simulink model "latestMPCforRTMapsGen"  (R2024a)
settings: Solver=FixedStepDiscrete  StartTime=0  StopTime=100  FixedStep=.05  RelTol=1e-3
undefined symbols (not defined in the file or in its folder): act_t_delay, aero_const, delta_U_max, delta_U_min, driver_set_spd, m, N, Qbar, Rbar, simStepSize, U_max, U_min, y_max, Y_min
settings Model: PacingRate=10  Creator=darkh  LastModifiedBy=darkh
settings DataIOCC: ReturnWorkspaceOutputsName=sltest_internal_rrSimulationOutputVariable
settings OptimizationCC: ZeroExternalMemoryAtStartup=off  ZeroInternalMemoryAtStartup=off
settings DebuggingCC: AlgebraicLoopMsg=none
settings RTWCC: Description=Generate an RTMaps component embedding the model  SystemTargetFile=rtmaps.tlc  TemplateMakefile=rtmaps_default_tmf  PostCodeGenCommand=rtmaps_post_code_generation(buildInfo)  RetainRTWFile=on  TargetLang=C++  GPUComputeCapability=3.5
settings STFCustomTargetCC: TargetLangStandard=C++11 (ISO)  ModelReferenceCompliant=off  ConcurrentExecutionCompliant=on  CombineOutputUpdateFcns=on  CodeInterfacePackaging=C++ class  CPPClassGenCompliant=on  GRTInterface=off  UseToolchainInfoCompliant=off  SystemTargetFile=rtmaps.tlc
settings GRTTargetCC: TargetLangStandard=C++11 (ISO)  ModelReferenceCompliant=off  ParMdlRefBuildCompliant=off  CompOptLevelCompliant=off  MatFileLogging=off  CodeInterfacePackaging=C++ class  UseToolchainInfoCompliant=off
settings ConfigComp: CovSaveName=sltest_covdata  CovMetricSettings=dcmwe  CovEnableCumulative=off  CovSaveSingleToWorkspaceVar=on  CovSaveOutputData=off

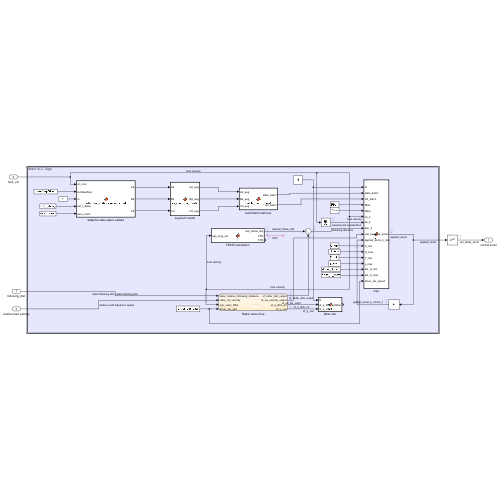
[thumbnail: Simulink's stored preview of the top-level diagram]
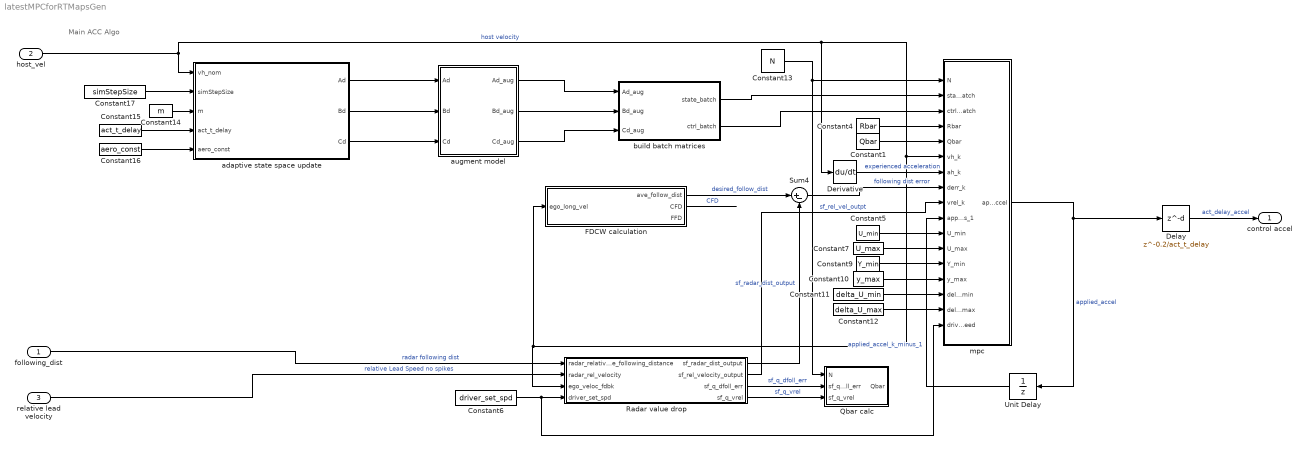
== system latestMPCforRTMapsGen ==
  note: Main ACC Algo
  following_dist : Inport
  host_vel : Inport  Port=2
  relative lead velocity : Inport  Port=3
  Constant1 : Constant  Value=Qbar
  Constant10 : Constant  Value=y_max
  Constant11 : Constant  Value=delta_U_min
  Constant12 : Constant  Value=delta_U_max
  Constant13 : Constant  Value=N
  Constant14 : Constant  Value=m
  Constant15 : Constant  Value=act_t_delay
  Constant16 : Constant  Value=aero_const
  Constant17 : Constant  Value=simStepSize
  Constant4 : Constant  Value=Rbar
  Constant5 : Constant  Value=U_min
  Constant6 : Constant  Value=driver_set_spd
  Constant7 : Constant  Value=U_max
  Constant9 : Constant  Value=Y_min
  Delay : Delay  DelayLength=0.2/act_t_delay
  Derivative : Derivative
  FDCW calculation : MATLAB Function  TreatAsAtomicUnit=on
  Qbar calc : MATLAB Function  TreatAsAtomicUnit=on  SystemSampleTime=simStepSize
  Radar value drop : Stateflow chart  TreatAsAtomicUnit=on
  Sum4 : Sum  Inputs=|+-
  Unit Delay : UnitDelay  SampleTime=-1  HasFrameUpgradeWarning=on
  adaptive state space update : MATLAB Function  TreatAsAtomicUnit=on
  augment model : MATLAB Function  TreatAsAtomicUnit=on
  build batch matrices : MATLAB Function  TreatAsAtomicUnit=on  SystemSampleTime=simStepSize
  mpc : MATLAB Function  TreatAsAtomicUnit=on  SystemSampleTime=simStepSize
  control accel : Outport
  wires:
  host_vel/1 -> adaptive state space update/1(vh_nom), Derivative/1, FDCW calculation/1(ego_long_vel), Radar value drop/3(ego_veloc_fdbk), mpc/6(vh_k)  "host velocity"
  Sum4/1 -> mpc/8(derr_k)  "following dist error"
  relative lead velocity/1 -> Radar value drop/2(radar_rel_velocity)  "relative Lead Speed no spikes"
  FDCW calculation/1(ave_follow_dist) -> Sum4/1  "desired_follow_dist"
  FDCW calculation/2(CFD) -> ?  "CFD"
  following_dist/1 -> Radar value drop/1(radar_relative_following_distance)  "radar following dist"
  Derivative/1 -> mpc/7(ah_k)  "experienced acceleration"
  Constant4/1 -> mpc/4(Rbar)
  Radar value drop/1(sf_radar_dist_output) -> Sum4/2  "sf_radar_dist_output"
  Constant6/1 -> mpc/17(driver_set_speed), Radar value drop/4(driver_set_spd)
  Radar value drop/2(sf_rel_velocity_output) -> mpc/9(vrel_k)  "sf_rel_vel_outpt"
  Radar value drop/3(sf_q_dfoll_err) -> Qbar calc/2(sf_q_dfoll_err)  "sf_q_dfoll_err"
  Radar value drop/4(sf_q_vrel) -> Qbar calc/3(sf_q_vrel)  "sf_q_vrel"
  Unit Delay/1 -> mpc/10(applied_accel_k_minus_1)  "applied_accel_k_minus_1"
  Constant5/1 -> mpc/11(U_min)
  Constant7/1 -> mpc/12(U_max)
  Constant9/1 -> mpc/13(Y_min)
  Constant10/1 -> mpc/14(y_max)
  Constant11/1 -> mpc/15(del_U_min)
  Constant12/1 -> mpc/16(del_U_max)
  Constant1/1 -> mpc/5(Qbar)
  mpc/1(applied_accel) -> Unit Delay/1, Delay/1  "applied_accel"
  Constant14/1 -> adaptive state space update/3(m)
  Constant15/1 -> adaptive state space update/4(act_t_delay)
  Constant16/1 -> adaptive state space update/5(aero_const)
  Constant17/1 -> adaptive state space update/2(simStepSize)
  augment model/3(Cd_aug) -> build batch matrices/3(Cd_aug)
  augment model/2(Bd_aug) -> build batch matrices/2(Bd_aug)
  augment model/1(Ad_aug) -> build batch matrices/1(Ad_aug)
  Constant13/1 -> Qbar calc/1(N), mpc/1(N)
  adaptive state space update/1(Ad) -> augment model/1(Ad)
  adaptive state space update/2(Bd) -> augment model/2(Bd)
  adaptive state space update/3(Cd) -> augment model/3(Cd)
  Delay/1 -> control accel/1  "act_delay_accel"
  build batch matrices/1(state_batch) -> mpc/2(state_batch)
  build batch matrices/2(ctrl_batch) -> mpc/3(ctrl_batch)

== matlab function latestMPCforRTMapsGen/build batch matrices ==
  data: state_batch output; Ad_aug input; Bd_aug input; Cd_aug input; ctrl_batch output
function [state_batch,ctrl_batch] = batch_matrix_build(Ad_aug,Bd_aug,Cd_aug)
[ny1,ny2] = size(Cd_aug);
[~,nu] = size(Bd_aug);

N=20;

% Building batch matrices for MPC prediction of output states
% batch matrix for state vector
state_batch = zeros(N*ny1, ny2);
for i = 1:N
    state_batch((i-1)*ny1+1 : i*ny1, :) = Cd_aug*(Ad_aug^i);
end

% Batch matrix for control vector
ctrl_batch = zeros(N*ny1, N*nu); % pre-allocate, fixed size

Apow = eye(size(Ad_aug)); % A^0
for i = 1:N
    % first column block for row i
    ctrl_batch((i-1)*ny1+(1:ny1), 1:nu) = Cd_aug*Apow*Bd_aug;
    % copy to the right for j = 2…i
    col = nu; % offset for next column
    Apow_j = Apow;
    for j = 2:i
        Apow_j = Apow_j / Ad_aug; % A^(i-j) (cheaper than repeated power)
        ctrl_batch((i-1)*ny1+(1:ny1), (j-1)*nu+(1:nu)) = Cd_aug*Apow_j*Bd_aug;
        col = col + nu;
    end
    Apow = Apow*Ad_aug; % advance A^i
end

== matlab function latestMPCforRTMapsGen/FDCW calculation ==
  settings: updateMethod=DISCRETE
  data: ego_long_vel input; ave_follow_dist output; CFD output; FFD output
% Function to determine the closest (CFD) and furthest follow distance (FFD) for the
% ego vehicle relative to the lead vehicle given the ego vehicle's current
% velocity

% This function outputs the middle distance value between the CFD and FFD
% and those values respectively as well

function [ave_follow_dist, CFD, FFD] = fcn(ego_long_vel)
    persistent dist_history window_size smoothing_weights
    
    % Initialize (first call only)
    if isempty(dist_history)
        window_size = 5;  % Number of past samples
        dist_history = zeros(1, window_size);
        
        % Define and normalize weights (e.g., linear decay)
        smoothing_weights = linspace(1, 0.5, window_size);  % Weights from 1.0 to 0.5
        smoothing_weights = smoothing_weights / sum(smoothing_weights);  % Normalize
    end
    ego_long_vel_mph = ego_long_vel*2.23694;
    
    if ego_long_vel_mph > 0 && ego_long_vel_mph < 20
        CFD = 2.8*ego_long_vel_mph^0.45+8;
        FFD = 100-0.2*(20-ego_long_vel_mph)^2;
    elseif ego_long_vel_mph <= 0
        CFD = 8;
        FFD = 100-0.2*(20)^2;
    else
        CFD = 2.8*ego_long_vel_mph^0.45+8;
        FFD = 100;
    end
    AveFollowDist_Gain = 3;


    % --- Update history buffer ---
    dist_history = [ ((AveFollowDist_Gain-1)*CFD + FFD)/AveFollowDist_Gain , dist_history(1:end-1)];  % FIFO

    % --- Smoothed average (weighted, normalized) ---
    smoothed_ave_dist = sum(dist_history .* smoothing_weights);
    
    % --- Clamp to CFD/FFD bounds ---
    ave_follow_dist = min(max(smoothed_ave_dist, CFD), FFD);
end

== matlab function latestMPCforRTMapsGen/adaptive state space update ==
  data: vh_nom input; simStepSize input; Ad output; m input; act_t_delay input; aero_const input; Bd output; Cd output
function [Ad,Bd,Cd] = adaptive_state_space_model(vh_nom, simStepSize, m, act_t_delay, aero_const)
% multiplying A matrix term with current vehicle velocity vh_nom to update
% state space model for adaptive MPC
Ac = [0,1,0,0; -aero_const*vh_nom/(m*act_t_delay), -1/act_t_delay, 0,0;0,0,0,-1;0,-1,0,0]; % with drag term
% Ac = [0,1,0,0; 0, -1/act_t_delay, 0,0;0,0,0,-1;0,-1,0,0]; % without the velocity dependent drag term
Bc = [0;1/act_t_delay;0;0];

% Using Euler discretization to obtain the discrete time matrices from the continuous time system
Ad = eye(4) + Ac.*simStepSize;
Bd = Bc.*simStepSize;
Cd = eye(4);

== matlab function latestMPCforRTMapsGen/mpc ==
  data: N input; state_batch input; ctrl_batch input; Rbar input; Qbar input; applied_accel output; vh_k input; ah_k input; derr_k input; vrel_k input; applied_accel_k_minus_1 input; U_min input; U_max input; Y_min input; y_max input; del_U_min input; del_U_max input; driver_set_speed input
function applied_accel  = mpc(N, state_batch, ctrl_batch, Rbar, Qbar, vh_k, ah_k, derr_k, vrel_k, applied_accel_k_minus_1, U_min, U_max, Y_min, y_max, del_U_min, del_U_max, driver_set_speed)
% Defining MPC and system variables
num_outpts = 4
num_ctrl = 1;

state_vec_curr = [vh_k, ah_k, derr_k, vrel_k, applied_accel_k_minus_1]';

H = 2*(ctrl_batch' * Qbar * ctrl_batch + Rbar); % symmetric Hessian
% tiny regulariser to ensure positive-definite
H = (H+H.')/2 + 1e-8*eye(size(H));

f = 2*(ctrl_batch' * Qbar * state_batch * state_vec_curr);

persistent del_Uopt_k_minus_1 % defining persistent variable to keep track of computed optimal control signal from previous iteration
if isempty(del_Uopt_k_minus_1)
    % del_Uopt_k_minus_1 = [0,0,0,0,0,0,0,0,0,0]'; % for N = 10
    del_Uopt_k_minus_1 = [0,0,0,0,0,0,0,0,0,0,0,0,0,0,0,0,0,0,0,0]'; % for N = 20
end

%% Defining the control input limits on delta_u based on limits on u

% Determining U(k-1) from the previous control signal u(k-1) and the previous full predicted control signal delta_Uopt(k-1)
Ubar_k_minus_1 = zeros(N*num_ctrl, 1); % Initializing
Ubar_k_minus_1(1:num_ctrl,:) = applied_accel_k_minus_1; % Populating the first control vector in Uopt(k-1) as u(k-1) = [accel_app(k-1)]'

for i = 1:N-1
    Ubar_k_minus_1(i*num_ctrl+1 : (i+1)*num_ctrl, :) = Ubar_k_minus_1((i-1)*num_ctrl+1 : i*num_ctrl, :) + del_Uopt_k_minus_1(i*num_ctrl+1 : (i+1)*num_ctrl, :); % performing u(k) = u(k-1) + delta_u(k-1) for all elements to populate Uopt(k-1)
end

% Defining the maximum output limit Y_max since the driver set speed may change
Y_max = zeros(N*num_outpts, 1);
for i = 1:N
    Y_max((i-1)*num_outpts + 1: i*num_outpts,:) = [driver_set_speed;y_max];
end

% Constraints on input: applied acceleration
A_qp_inpts = [eye(num_ctrl*N); -eye(num_ctrl*N)]; % both lower and upper acceleration bounds for inputs
b_qp_inpts = [U_max - Ubar_k_minus_1; -U_min + Ubar_k_minus_1];

% A_qp_inpts = [-eye(num_ctrl*N)];  % only lower bounds for inputs
% b_qp_inpts = [-U_min + Ubar_k_minus_1];

% Constraints on feeoutputs vh, ah, dfoll_err, vrel
A_qp_otpts = [ctrl_batch;-ctrl_batch]; % Both upper and lower bounds for outputs
b_qp_otpts = [Y_max - state_batch*state_vec_curr; -Y_min + state_batch*state_vec_curr];

% A_qp_otpts = [-ctrl_batch]; % only lower bounds for outputs
% b_qp_otpts = [-Y_min + state_batch*state_vec_curr];

A_qp = [A_qp_inpts; A_qp_otpts];
b_qp = [b_qp_inpts; b_qp_otpts]; 

% code where quadprog is used to solve the optimization problem
options = optimoptions('quadprog','Algorithm','active-set'); % options for quadprog
delta_Uopt = quadprog(H,f,A_qp,b_qp,[],[],del_U_min,del_U_max,del_Uopt_k_minus_1,options); % includes constraints on delta_u here

% code where mpcInteriorPointSolver is used to solve the optimization problem
% options = mpcInteriorPointOptions; % options for mpcInteriorPointSolver
% delta_Uopt = mpcInteriorPointSolver(H,f,A_qp,b_qp,zeros(0,N*num_ctrl),zeros(0,1),del_Uopt_k_minus_1,options); % does not include constraints on delta_u here

del_Uopt_k_minus_1 = delta_Uopt; % saving computed control signal for optimal delta U (over prediction horizon) for use in next iteration; becomes next delta_Uopt(k-1)

delta_u_apply = delta_Uopt(1:num_ctrl,:); % nu = number of inputs; receding horizon so only selecting the first control vector in collection to apply to plant

applied_accel = applied_accel_k_minus_1 + delta_u_apply; % Adding to previous control input since state space model is augmented to determine delta_u

== stateflow chart latestMPCforRTMapsGen/Radar value drop ==
  state Radar_State_Lead_Veh_Present_and_Detected
    sf_radar_dist_output = radar_relative_following_distance;
    sf_rel_velocity_output = radar_rel_velocity;
    sf_q_dfoll_err = 100;
    sf_q_vrel = 100;
  state Output_Spoof_To_Keep_Moving
    sf_radar_dist_output = 100;
    set_spd_err = driver_set_spd - ego_veloc_fdbk;
    sf_rel_velocity_output = set_spd_err;
    sf_q_dfoll_err = 0;
    sf_q_vrel = 40;
  (default) -> Radar_State_Lead_Veh_Present_and_Detected
  Radar_State_Lead_Veh_Present_and_Detected -> Output_Spoof_To_Keep_Moving : [radar_relative_following_distance == 0 && radar_rel_velocity < 0.9]
  Output_Spoof_To_Keep_Moving -> Radar_State_Lead_Veh_Present_and_Detected : [radar_relative_following_distance > 0]
  data: radar_relative_following_distance input; sf_radar_dist_output output; radar_rel_velocity input; ego_veloc_fdbk input; sf_rel_velocity_output output; driver_set_spd input; set_spd_err local; sf_q_dfoll_err output; sf_q_vrel output

== matlab function latestMPCforRTMapsGen/Qbar calc ==
  data: N input; sf_q_dfoll_err input; Qbar output; sf_q_vrel input
function Qbar = fcn(N, sf_q_dfoll_err, sf_q_vrel) 
    N = 5;
    q_vh = 0;
    q_ah = 20;
    % q_dfoll = 1000; % Set from stateflow
    % q_vrel = 100;
    
    Q = diag([q_vh, q_ah, sf_q_dfoll_err, sf_q_vrel]);
    Qbar = kron(eye(N),Q);

== matlab function latestMPCforRTMapsGen/augment model ==
  data: Ad input; Ad_aug output; Bd input; Cd input; Bd_aug output; Cd_aug output
function [Ad_aug,Bd_aug,Cd_aug] = augment_ss_model(Ad,Bd,Cd)
[num_states,~] = size(Ad); % number of states in unaugmented system model
[~,num_ctrl] = size(Bd); % number of control inputs to system
[num_outpts,~] = size(Cd); % number of outputs from system

% Augmenting the State space model to have control vector delta_u and new state vec [x(k)', u(k-1)]' and output vec y(k) = x(k) 
Ad_aug = [Ad, Bd; zeros([num_ctrl num_states]), eye(num_ctrl)];
Bd_aug = [Bd; eye(num_ctrl)];
Cd_aug = [Cd, zeros([num_outpts num_ctrl])];
